simulink model "SMA_displacementIn_PC2_4"  (R2018a)
settings: Solver=ode15s  StartTime=0.0  StopTime=100  RelTol=1e-8  AbsTol=1e-8  EnableMultiTasking=on
values from neighbouring files (symbols this model uses):
  param_b = 10    [plot_task_4.m]
  param_factor = 0.0137    [plot_task_4.m]
  param_J = params_PC2.alpha * 2 * pi * params_PC2.r0 * params_PC2.L0 * param_N * params_PC2.delta_T    [plot_task_4.m]
  param_J0_yin = 0.7845    [plot_task_4.m]
  param_k = 500    [plot_task_4.m]
  param_m = 0.3    [plot_task_4.m]
  param_N = 20    [plot_task_4.m]
  params_PC2 = struct    [Parameter_PC2.m]
settings Model: Creator=Gianluca  LastModifiedBy=tim
settings SolverCC: AutoScaleAbsTol=off
settings DataIOCC: LimitDataPoints=on  SaveFormat=Array
settings OptimizationCC: LifeSpan=inf
settings DebuggingCC: UnderspecifiedInitializationDetection=Classic  MergeDetectMultiDrivingBlocksExec=none  SolverPrmCheckMsg=warning  StateNameClashWarn=warning  SFUnexpectedBacktrackingDiag=warning  SFNoUnconditionalDefaultTransitionDiag=warning  SFExecutionAtInitializationDiag=none
settings HardwareCC: ProdBitPerPointer=32  ProdBitPerSizeT=32  ProdBitPerPtrDiffT=32  ProdLargestAtomicFloat=None  ProdIntDivRoundTo=Undefined  ProdEndianess=Unspecified  ProdWordSize=32  ProdHWDeviceType=32-bit Generic
settings ModelReferenceCC: PropagateSignalLabelsOutOfModel=off
settings CodeAppCC: StateflowObjectComments=on
settings GRTTargetCC: TargetLangStandard=C89/C90 (ANSI)  GeneratePreprocessorConditionals=Disable all
settings ConfigComp: CovMetricSettings=dw  CovHtmlReporting=on  CovSaveCumulativeToWorkspaceVar=on  CovSaveSingleToWorkspaceVar=on  CovExternalEMLEnable=off

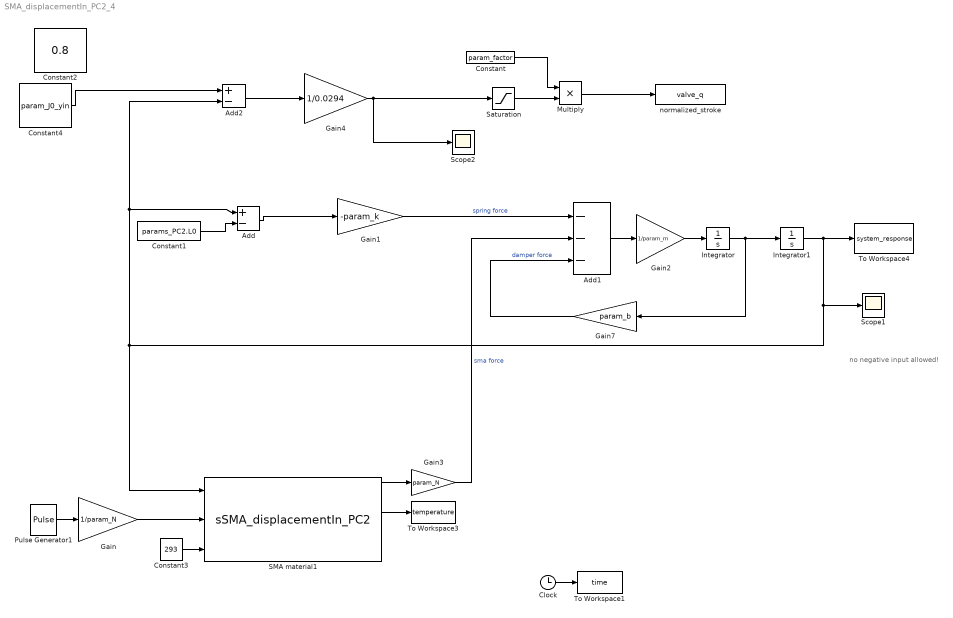
== system SMA_displacementIn_PC2_4 ==
  note: no negative input allowed!
  Add : Sum  Inputs=+-
  Add1 : Sum  Inputs=---
  Add2 : Sum  Inputs=+-
  Clock : Clock
  Constant : Constant  Value=param_factor
  Constant1 : Constant  Value=params_PC2.L0
  Constant2 : Constant  Value=0.8
  Constant3 : Constant  Value=293
  Constant4 : Constant  Value=param_J0_yin
  Gain : Gain  Gain=1/param_N
  Gain1 : Gain  Gain=-param_k
  Gain2 : Gain  Gain=1/param_m
  Gain3 : Gain  Gain=param_N
  Gain4 : Gain  Gain=1/0.0294
  Gain7 : Gain  Gain=param_b
  Integrator : Integrator
  Integrator1 : Integrator  InitialCondition=param_J0_yin
  Multiply : Product
  Pulse Generator1 : DiscretePulseGenerator  PulseType=Time based  Amplitude=param_J  Period=10  PulseWidth=50
  SMA material1 : M-S-Function  FunctionName=sSMA_displacementIn_PC2  Parameters=params_PC2, initConds_PC2
      mask Display:
      | color('black');
      | patch(3*[-1 1 1 -1],1.1*[-1 -1 1 1],[1 1 1]);
      | patch([-1.6 -0.8],[-0.9 0.3],[0 0 0]);
      | patch([-0.8 1.2],[0.3 0.3],[0 0 0]);
      | patch([1.6 0.8],[0.9 -0.3],[0 0 0]);
      | patch([0.8 -1.2],[-0.3 -0.3],[0 0 0]);
      | disp('SMA');
      | 
      | color('blue');
      | port_label('input', 1, 'y [m]','texmode','on');
      | port_label('input', 2, 'J [W]','texmode','on');
      | port_label('input', 3, 'T_E [K]','texmode','on');
      | 
      | color('red');
      | port_label('output', 1, 'F [N]','texmode','on');
      | port_label('output', 2, 'x_+, x_-, x_A [-]','texmode','on');
      | port_label('output', 3, 'T [K]','texmode','on');
      | port_label('output', 4, '\epsilon [-]','texmode','on');
      | port_label('output', 5, '\sigma [Pa]','texmode','on');
      | port_label('output', 6, 'R [\Omega]','texmode','on');
  Saturation : Saturate  UpperLimit=1  LowerLimit=0
  Scope1 : Scope
  Scope2 : Scope
  To Workspace1 : ToWorkspace  VariableName=time  SampleTime=-1
  To Workspace3 : ToWorkspace  VariableName=temperature  SampleTime=-1
  To Workspace4 : ToWorkspace  VariableName=system_response  SampleTime=-1
  normalized_stroke : ToWorkspace  VariableName=valve_q  SampleTime=-1
  wires:
  Gain7/1 -> Add1/3  "damper force"
  Integrator/1 -> Integrator1/1, Gain7/1
  Gain3/1 -> Add1/2  "sma force"
  Pulse Generator1/1 -> Gain/1
  Constant3/1 -> SMA material1/3
  SMA material1/1 -> Gain3/1
  SMA material1/3 -> To Workspace3/1
  Gain/1 -> SMA material1/2
  Gain1/1 -> Add1/1  "spring force"
  Add1/1 -> Gain2/1
  Gain2/1 -> Integrator/1
  Gain4/1 -> Saturation/1, Scope2/1
  Add2/1 -> Gain4/1
  Integrator1/1 -> To Workspace4/1, Add/1, Add2/2, SMA material1/1, Scope1/1
  Add/1 -> Gain1/1
  Clock/1 -> To Workspace1/1
  Constant1/1 -> Add/2
  Constant4/1 -> Add2/1
  Constant/1 -> Multiply/1
  Multiply/1 -> normalized_stroke/1
  Saturation/1 -> Multiply/2
